simulink model "EE405L_Lab4"  (R2021b)
settings: Solver=VariableStepAuto  StartTime=0.0  StopTime=20  RelTol=1e-3
libraries: simulink x3
settings Model: Creator=Kevin  LastModifiedBy=Kevin

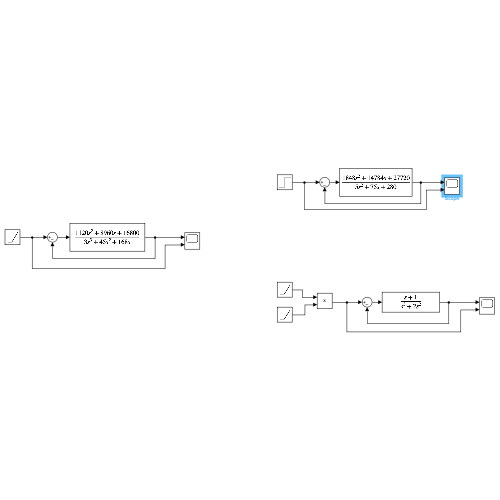
[thumbnail: Simulink's stored preview of the top-level diagram]
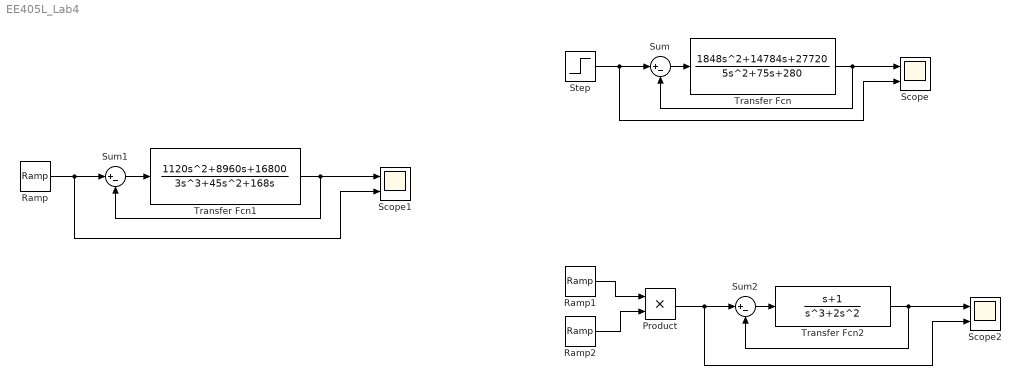
== system EE405L_Lab4 ==
  Product : Product
  Ramp : simulink/Sources/Ramp  slope=1  start=0  InitialOutput=0
  Ramp1 : simulink/Sources/Ramp  slope=1  start=0  InitialOutput=0
  Ramp2 : simulink/Sources/Ramp  slope=1  start=0  InitialOutput=0
  Scope : Scope  NumInputPorts=2
  Scope1 : Scope  NumInputPorts=2
  Scope2 : Scope  NumInputPorts=2
  Step : Step  SampleTime=0
  Sum : Sum  Inputs=|+-
  Sum1 : Sum  Inputs=|+-
  Sum2 : Sum  Inputs=|+-
  Transfer Fcn : TransferFcn  Numerator=[1848 14784 27720]  Denominator=[5 75 280]
  Transfer Fcn1 : TransferFcn  Numerator=[1120 8960 16800]  Denominator=[3 45 168 0]
  Transfer Fcn2 : TransferFcn  Numerator=[1 1]  Denominator=[1 2 0 0]
  wires:
  Sum/1 -> Transfer Fcn/1
  Transfer Fcn/1 -> Scope/1, Sum/2
  Step/1 -> Scope/2, Sum/1
  Ramp/1 -> Scope1/2, Sum1/1
  Transfer Fcn1/1 -> Sum1/2, Scope1/1
  Sum1/1 -> Transfer Fcn1/1
  Product/1 -> Scope2/2, Sum2/1
  Transfer Fcn2/1 -> Scope2/1, Sum2/2
  Sum2/1 -> Transfer Fcn2/1
  Ramp1/1 -> Product/1
  Ramp2/1 -> Product/2
